simulink model "p3_siso"  (R2021b)
settings: Solver=VariableStepAuto  StartTime=0.0  StopTime=10.0  RelTol=1e-3
libraries: cstblocks x3
settings Model: Creator=dabner  LastModifiedBy=dabner

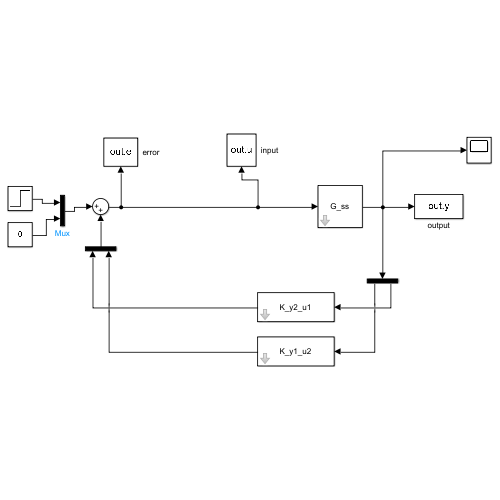
[thumbnail: Simulink's stored preview of the top-level diagram]
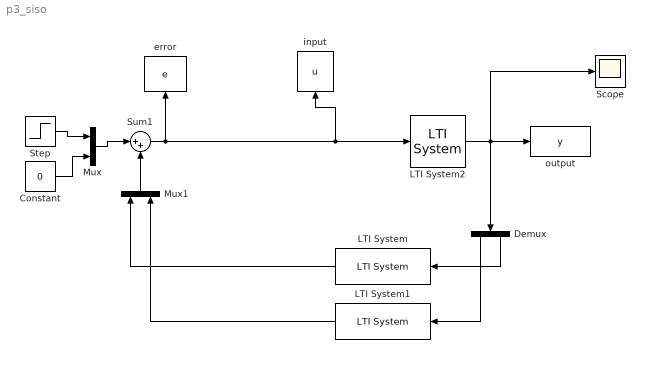
== system p3_siso ==
  Constant : Constant  Value=0
  Demux : Demux  Outputs=2
  LTI System : cstblocks/LTI System  sys=K_y2_u1  IC=[]
  LTI System1 : cstblocks/LTI System  sys=K_y1_u2  IC=[]
  LTI System2 : cstblocks/LTI System  sys=G_ss  IC=[]
  Mux : Mux  Inputs=2
  Mux1 : Mux  Inputs=2
  Scope : Scope
  Step : Step  SampleTime=0
  Sum1 : Sum  Inputs=|++
  error : ToWorkspace  VariableName=e  SampleTime=-1
  input : ToWorkspace  VariableName=u  SampleTime=-1
  output : ToWorkspace  VariableName=y  SampleTime=-1
  wires:
  Step/1 -> Mux/1
  Mux/1 -> Sum1/1
  Sum1/1 -> LTI System2/1, input/1, error/1
  LTI System2/1 -> Scope/1, Demux/1, output/1
  Constant/1 -> Mux/2
  Demux/2 -> LTI System/1
  Demux/1 -> LTI System1/1
  Mux1/1 -> Sum1/2
  LTI System1/1 -> Mux1/2
  LTI System/1 -> Mux1/1
